simulink model "test"  (R2013a)
settings: Solver=ode45  StartTime=0.0  StopTime=time  RelTol=1e-3
values from neighbouring files (symbols this model uses):
  b = 0.1    [init.m]    (also in pathPlotter.m = 0.025)
  eta_0 = [0,0,0,0,0,0]'    [init.m]
  g = 9.81    [init.m]
  I = diag([0.1, 0.1, 0.2])    [init.m]
  k = 3    [init.m]
  K_d = diag([-1,-1,-0.5])    [init.m]
  k_d = -20    [init.m]
  K_d_pos = 2*sqrt(K_p_pos(1,1))*eye(2)    [init.m]
  K_i = diag([0,0,0])    [init.m]
  k_i = 150    [init.m]
  K_i_pos = 0.05 * eye(2)    [init.m]
  K_p = diag([20,20,0.45])    [init.m]
  k_p = 100    [init.m]
  K_p_pos = 0.5*eye(2)    [init.m]
  l = 0.25    [init.m]
  m = 3    [init.m]
  nodePosition = [0.5,0.5,0]'    [init.m]
  nu_0 = [0,0,0,0,0,0]'    [init.m]
  pos_ref = [10,10,-10]'    [init.m]
  wind = [0.5,0]'    [init.m]
  windDir = 0    [init.m]
libraries: simulink x1
settings Model: Creator=vegardvo  LastModifiedBy=vegardvo

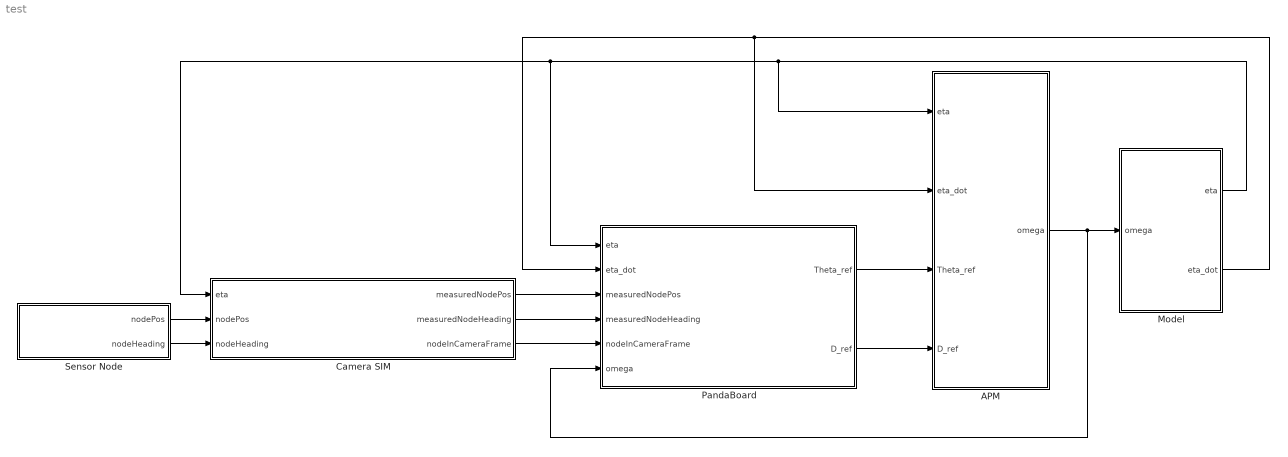
== system test ==
  APM : Subsystem
  Camera SIM : Subsystem
  Model : Subsystem
  PandaBoard : Subsystem
  Sensor Node : Subsystem
  wires:
  Sensor Node/1(nodePos) -> Camera SIM/2(nodePos)
  Sensor Node/2(nodeHeading) -> Camera SIM/3(nodeHeading)
  APM/1(omega) -> Model/1(omega), PandaBoard/6(omega)
  Model/1(eta) -> APM/1(eta), PandaBoard/1(eta), Camera SIM/1(eta)
  Model/2(eta_dot) -> APM/2(eta_dot), PandaBoard/2(eta_dot)
  Camera SIM/3(nodeInCameraFrame) -> PandaBoard/5(nodeInCameraFrame)
  Camera SIM/2(measuredNodeHeading) -> PandaBoard/4(measuredNodeHeading)
  Camera SIM/1(measuredNodePos) -> PandaBoard/3(measuredNodePos)
  PandaBoard/1(Theta_ref) -> APM/3(Theta_ref)
  PandaBoard/2(D_ref) -> APM/4(D_ref)

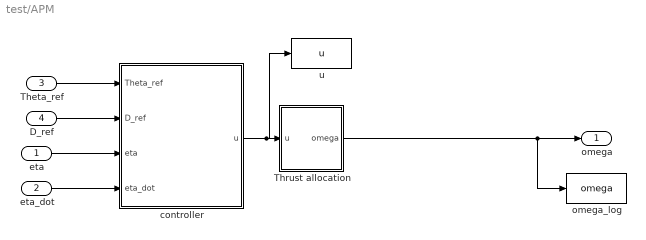
== system test/APM ==
  eta : Inport
  eta_dot : Inport  Port=2
  Theta_ref : Inport  Port=3
  D_ref : Inport  Port=4
  Thrust allocation : Subsystem
  controller : Subsystem
  omega_log : ToWorkspace  VariableName=omega  SampleTime=-1  SaveFormat=Timeseries
  u : ToWorkspace  VariableName=u  SampleTime=-1  SaveFormat=Timeseries
  omega : Outport
  wires:
  Thrust allocation/1(omega) -> omega/1, omega_log/1
  controller/1(u) -> u/1, Thrust allocation/1(u)
  D_ref/1 -> controller/2(D_ref)
  Theta_ref/1 -> controller/1(Theta_ref)
  eta/1 -> controller/3(eta)
  eta_dot/1 -> controller/4(eta_dot)

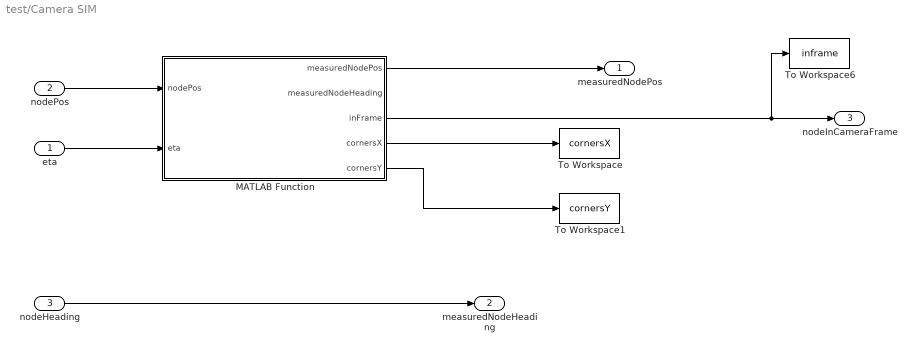
== system test/Camera SIM ==
  eta : Inport
  nodePos : Inport  Port=2
  nodeHeading : Inport  Port=3
  MATLAB Function : MATLAB Function  TreatAsAtomicUnit=on
  To Workspace : ToWorkspace  VariableName=cornersX  SampleTime=-1  SaveFormat=Timeseries
  To Workspace1 : ToWorkspace  VariableName=cornersY  SampleTime=-1  SaveFormat=Timeseries
  To Workspace6 : ToWorkspace  VariableName=inframe  SampleTime=-1  SaveFormat=Timeseries
  measuredNodePos : Outport
  measuredNodeHeading : Outport  Port=2
  nodeInCameraFrame : Outport  Port=3
  wires:
  nodePos/1 -> MATLAB Function/1(nodePos)
  MATLAB Function/1(measuredNodePos) -> measuredNodePos/1
  eta/1 -> MATLAB Function/2(eta)
  MATLAB Function/3(inFrame) -> To Workspace6/1, nodeInCameraFrame/1
  nodeHeading/1 -> measuredNodeHeading/1
  MATLAB Function/4(cornersX) -> To Workspace/1
  MATLAB Function/5(cornersY) -> To Workspace1/1

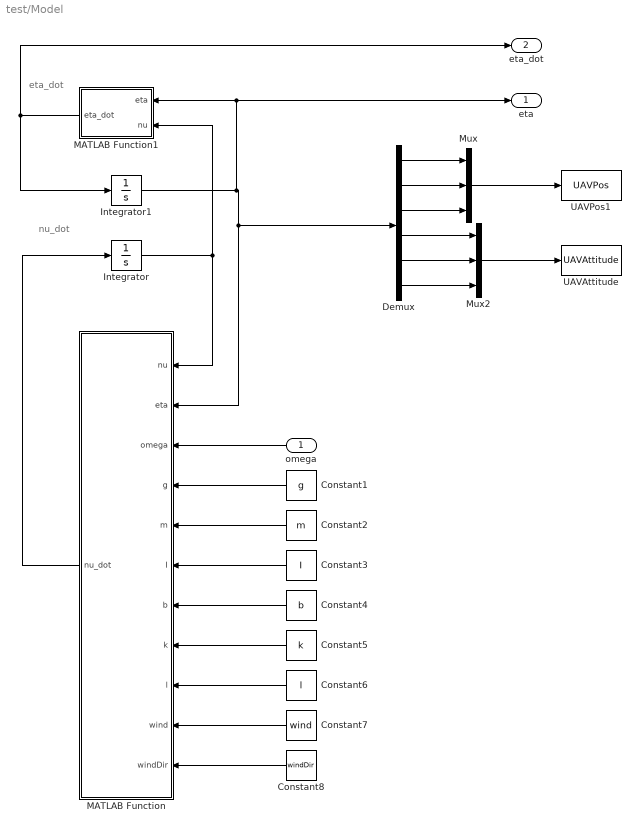
== system test/Model ==
  note: eta_dot
  note: nu_dot
  omega : Inport
  Constant1 : Constant  Value=g
  Constant2 : Constant  Value=m
  Constant3 : Constant  Value=I
  Constant4 : Constant  Value=b
  Constant5 : Constant  Value=k
  Constant6 : Constant  Value=l
  Constant7 : Constant  Value=wind
  Constant8 : Constant  Value=windDir
  Demux : Demux  Outputs=6
  Integrator : Integrator  InitialCondition=nu_0
  Integrator1 : Integrator  InitialCondition=eta_0
  MATLAB Function : MATLAB Function  TreatAsAtomicUnit=on
  MATLAB Function1 : MATLAB Function  TreatAsAtomicUnit=on
  Mux : Mux  Inputs=3
  Mux2 : Mux  Inputs=3
  UAVAttitude : ToWorkspace  VariableName=UAVAttitude  SampleTime=-1  SaveFormat=Timeseries
  UAVPos1 : ToWorkspace  VariableName=UAVPos  SampleTime=-1  SaveFormat=Timeseries
  eta : Outport
  eta_dot : Outport  Port=2
  wires:
  MATLAB Function/1(nu_dot) -> Integrator/1
  Integrator/1 -> MATLAB Function/1(nu), MATLAB Function1/2(nu)
  Integrator1/1 -> MATLAB Function/2(eta), Demux/1, MATLAB Function1/1(eta), eta/1
  Constant1/1 -> MATLAB Function/4(g)
  Constant2/1 -> MATLAB Function/5(m)
  Constant3/1 -> MATLAB Function/6(I)
  Demux/1 -> Mux/1
  Demux/2 -> Mux/2
  Demux/3 -> Mux/3
  Demux/4 -> Mux2/1
  Demux/5 -> Mux2/2
  Demux/6 -> Mux2/3
  Constant4/1 -> MATLAB Function/7(b)
  Constant5/1 -> MATLAB Function/8(k)
  Constant6/1 -> MATLAB Function/9(l)
  MATLAB Function1/1(eta_dot) -> Integrator1/1, eta_dot/1
  omega/1 -> MATLAB Function/3(omega)
  Mux/1 -> UAVPos1/1
  Mux2/1 -> UAVAttitude/1
  Constant8/1 -> MATLAB Function/11(windDir)
  Constant7/1 -> MATLAB Function/10(wind)

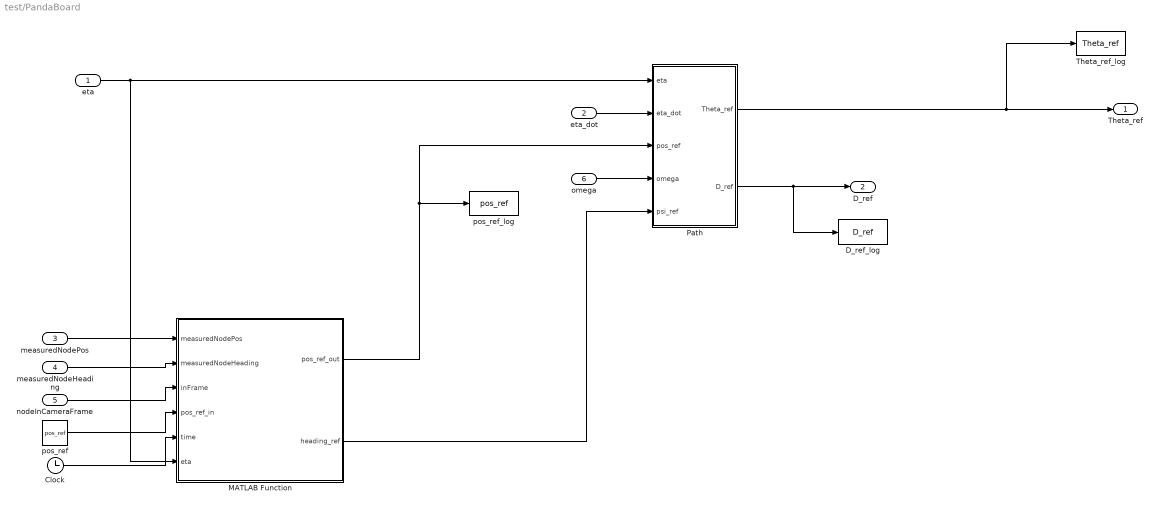
== system test/PandaBoard ==
  eta : Inport
  eta_dot : Inport  Port=2
  measuredNodePos : Inport  Port=3
  measuredNodeHeading : Inport  Port=4
  nodeInCameraFrame : Inport  Port=5
  omega : Inport  Port=6
  Clock : Clock
  D_ref_log : ToWorkspace  VariableName=D_ref  SampleTime=-1  SaveFormat=Timeseries
  MATLAB Function : MATLAB Function  TreatAsAtomicUnit=on
  Path : Subsystem
  Theta_ref_log : ToWorkspace  VariableName=Theta_ref  SampleTime=-1  SaveFormat=Timeseries
  pos_ref : Constant  Value=pos_ref
  pos_ref_log : ToWorkspace  VariableName=pos_ref  SampleTime=-1  SaveFormat=Timeseries
  Theta_ref : Outport
  D_ref : Outport  Port=2
  wires:
  Path/2(D_ref) -> D_ref/1, D_ref_log/1
  omega/1 -> Path/4(omega)
  eta_dot/1 -> Path/2(eta_dot)
  eta/1 -> MATLAB Function/6(eta), Path/1(eta)
  measuredNodePos/1 -> MATLAB Function/1(measuredNodePos)
  measuredNodeHeading/1 -> MATLAB Function/2(measuredNodeHeading)
  nodeInCameraFrame/1 -> MATLAB Function/3(inFrame)
  pos_ref/1 -> MATLAB Function/4(pos_ref_in)
  MATLAB Function/1(pos_ref_out) -> Path/3(pos_ref), pos_ref_log/1
  MATLAB Function/2(heading_ref) -> Path/5(psi_ref)
  Clock/1 -> MATLAB Function/5(time)
  Path/1(Theta_ref) -> Theta_ref_log/1, Theta_ref/1

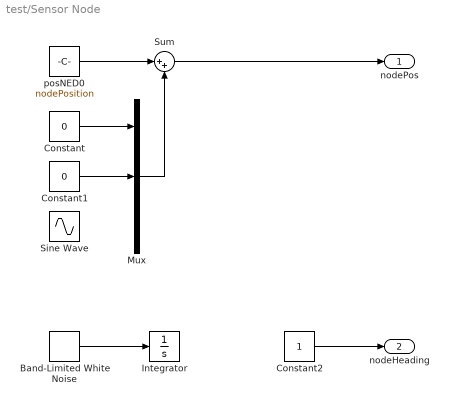
== system test/Sensor Node ==
  Band-Limited White Noise : simulink/Sources/Band-Limited White Noise  Cov=[0.1]  Ts=0.1  seed=[23341]
  Constant : Constant  Value=0
  Constant1 : Constant  Value=0
  Constant2 : Constant
  Integrator : Integrator
  Mux : Mux  Inputs=3
  Sine Wave : Sin  SampleTime=0
  Sum : Sum  Inputs=|++
  posNED0 : Constant  Value=nodePosition
  nodePos : Outport
  nodeHeading : Outport  Port=2
  wires:
  posNED0/1 -> Sum/1
  Sum/1 -> nodePos/1
  Mux/1 -> Sum/2
  Constant1/1 -> Mux/2
  Constant/1 -> Mux/1
  Band-Limited White Noise/1 -> Integrator/1
  Constant2/1 -> nodeHeading/1

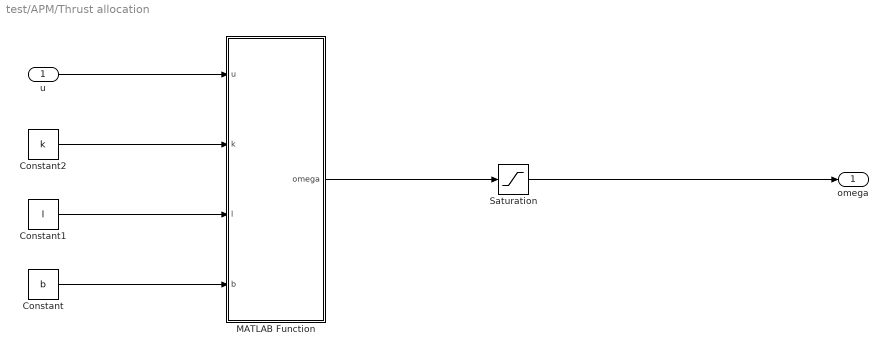
== system test/APM/Thrust allocation ==
  u : Inport
  Constant : Constant  Value=b
  Constant1 : Constant  Value=l
  Constant2 : Constant  Value=k
  MATLAB Function : MATLAB Function  TreatAsAtomicUnit=on
  Saturation : Saturate  UpperLimit=Inf  LowerLimit=0  ZeroCross=off
  omega : Outport
  wires:
  u/1 -> MATLAB Function/1(u)
  Constant2/1 -> MATLAB Function/2(k)
  Constant1/1 -> MATLAB Function/3(l)
  Constant/1 -> MATLAB Function/4(b)
  MATLAB Function/1(omega) -> Saturation/1
  Saturation/1 -> omega/1

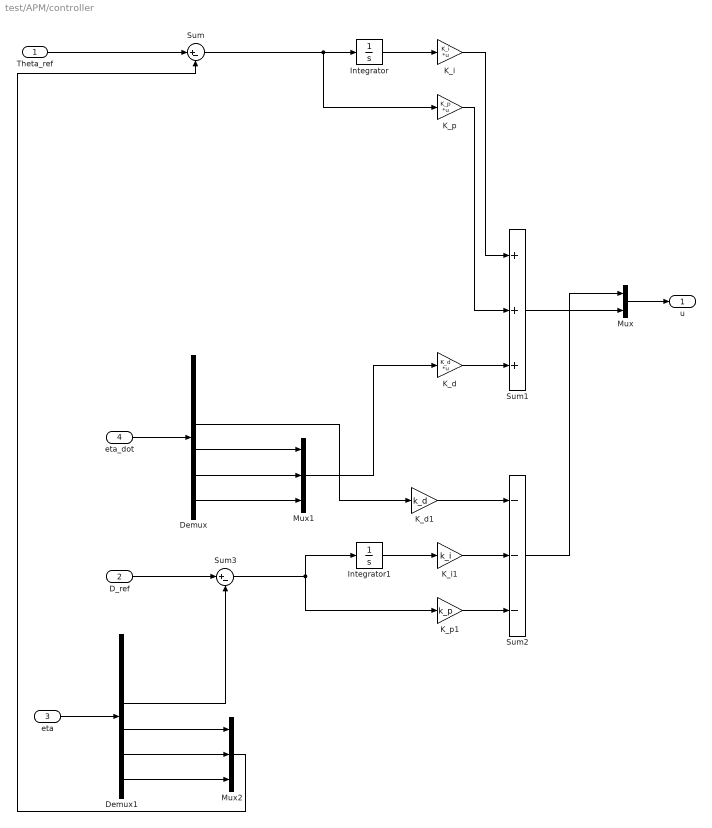
== system test/APM/controller ==
  Theta_ref : Inport
  D_ref : Inport  Port=2
  eta : Inport  Port=3
  eta_dot : Inport  Port=4
  Demux : Demux  Outputs=6
  Demux1 : Demux  Outputs=6
  Integrator : Integrator  InitialCondition=[0,0,0]'
  Integrator1 : Integrator
  K_d : Gain  Gain=K_d  Multiplication=Matrix(K*u)
  K_d1 : Gain  Gain=k_d
  K_i : Gain  Gain=K_i  Multiplication=Matrix(K*u)
  K_i1 : Gain  Gain=k_i
  K_p : Gain  Gain=K_p  Multiplication=Matrix(K*u)
  K_p1 : Gain  Gain=k_p
  Mux : Mux  Inputs=2
  Mux1 : Mux  Inputs=3
  Mux2 : Mux  Inputs=3
  Sum : Sum  Inputs=|+-
  Sum1 : Sum  Inputs=+++
  Sum2 : Sum  Inputs=---
  Sum3 : Sum  Inputs=|+-
  u : Outport
  wires:
  Sum/1 -> K_p/1, Integrator/1
  Integrator/1 -> K_i/1
  K_i/1 -> Sum1/1
  K_p/1 -> Sum1/2
  K_d/1 -> Sum1/3
  Integrator1/1 -> K_i1/1
  D_ref/1 -> Sum3/1
  Sum3/1 -> K_p1/1, Integrator1/1
  Mux/1 -> u/1
  eta_dot/1 -> Demux/1
  Mux1/1 -> K_d/1
  K_d1/1 -> Sum2/1
  eta/1 -> Demux1/1
  K_i1/1 -> Sum2/2
  K_p1/1 -> Sum2/3
  Sum2/1 -> Mux/1
  Sum1/1 -> Mux/2
  Demux1/3 -> Sum3/2
  Demux1/4 -> Mux2/1
  Demux1/5 -> Mux2/2
  Demux1/6 -> Mux2/3
  Mux2/1 -> Sum/2
  Demux/4 -> Mux1/1
  Demux/5 -> Mux1/2
  Demux/6 -> Mux1/3
  Demux/3 -> K_d1/1
  Theta_ref/1 -> Sum/1

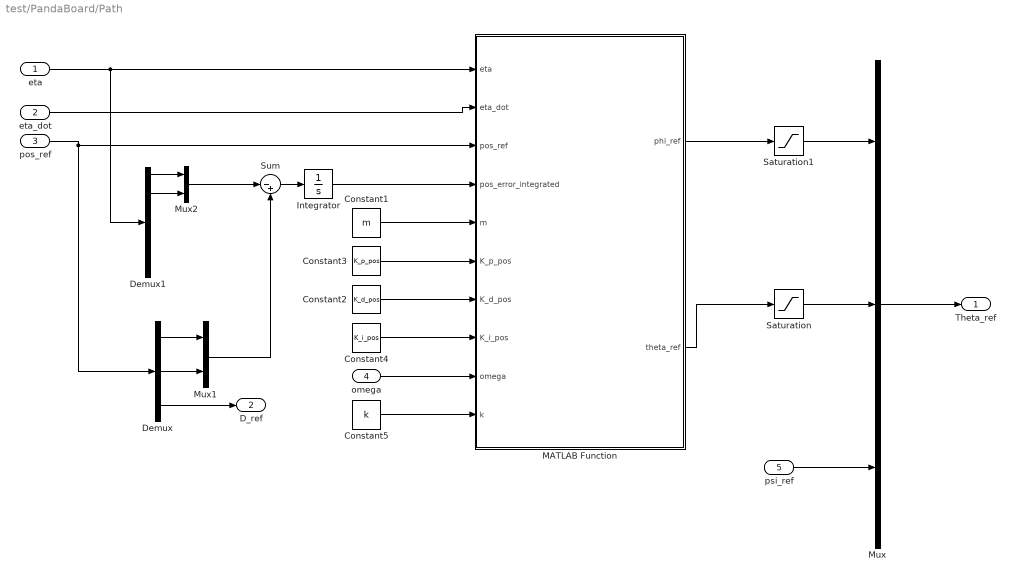
== system test/PandaBoard/Path ==
  eta : Inport
  eta_dot : Inport  Port=2
  pos_ref : Inport  Port=3
  omega : Inport  Port=4
  psi_ref : Inport  Port=5
  Constant1 : Constant  Value=m
  Constant2 : Constant  Value=K_d_pos
  Constant3 : Constant  Value=K_p_pos
  Constant4 : Constant  Value=K_i_pos
  Constant5 : Constant  Value=k
  Demux : Demux  Outputs=3
  Demux1 : Demux  Outputs=6
  Integrator : Integrator  LimitOutput=on  UpperSaturationLimit=100  LowerSaturationLimit=-100
  MATLAB Function : MATLAB Function  TreatAsAtomicUnit=on
  Mux : Mux  Inputs=3
  Mux1 : Mux  Inputs=2
  Mux2 : Mux  Inputs=2
  Saturation : Saturate  UpperLimit=0.2  LowerLimit=-0.2  ZeroCross=off
  Saturation1 : Saturate  UpperLimit=0.2  LowerLimit=-0.2  ZeroCross=off
  Sum : Sum  Inputs=|-+
  Theta_ref : Outport
  D_ref : Outport  Port=2
  wires:
  Mux/1 -> Theta_ref/1
  eta/1 -> Demux1/1, MATLAB Function/1(eta)
  pos_ref/1 -> MATLAB Function/3(pos_ref), Demux/1
  Demux/3 -> D_ref/1
  eta_dot/1 -> MATLAB Function/2(eta_dot)
  Constant1/1 -> MATLAB Function/5(m)
  Constant3/1 -> MATLAB Function/6(K_p_pos)
  Constant2/1 -> MATLAB Function/7(K_d_pos)
  MATLAB Function/1(phi_ref) -> Saturation1/1
  MATLAB Function/2(theta_ref) -> Saturation/1
  Saturation1/1 -> Mux/1
  Saturation/1 -> Mux/2
  psi_ref/1 -> Mux/3
  omega/1 -> MATLAB Function/9(omega)
  Constant5/1 -> MATLAB Function/10(k)
  Constant4/1 -> MATLAB Function/8(K_i_pos)
  Integrator/1 -> MATLAB Function/4(pos_error_integrated)
  Sum/1 -> Integrator/1
  Demux/1 -> Mux1/1
  Demux/2 -> Mux1/2
  Demux1/1 -> Mux2/1
  Demux1/2 -> Mux2/2
  Mux2/1 -> Sum/1
  Mux1/1 -> Sum/2

== matlab function test/APM/Thrust allocation/MATLAB Function ==
  data: u input; omega output; k input; l input; b input
function omega = fcn(u, k, l, b)
%#codegen

A = [k, k, k, k, k, k;
     -0.5*k*l, 0.5*k*l, k*l, 0.5*k*l, -0.5*k*l, -k*l;
     sqrt(3)/2*k*l, sqrt(3)/2*k*l, 0, -sqrt(3)/2*k*l, -sqrt(3)/2*k*l, 0;
     b, -b, b, -b, b, -b];

 A_pseudo = A'/(A*A');

omega = A_pseudo*u;
%omega = [1,1,1,1,1,1]';

== matlab function test/Model/MATLAB Function ==
  data: nu input; nu_dot output; eta input; omega input; g input; m input; I input; b input; k input; l input; wind input; windDir input
function nu_dot = fcn(nu, eta, omega, g, m, I, b, k, l, wind, windDir)
%#codegen

omega_squared = omega;%omega.^2;

M_rb = [m * eye(3), zeros(3);
        zeros(3)  , I];
 
%C_rb = [m*Smtrx(nu(4:6)), zeros(3);
%       zeros(3), -Smtrx(I*nu(4:6))];
   
C_rb = m2c(M_rb, nu);

RotWind = [cos(windDir), sin(windDir);
          -sin(windDir), cos(windDir)];
wind_b = RotWind * wind;

tau_b = [-m*g*sin(eta(5)) + wind_b(1);
       m*g*cos(eta(5))*sin(eta(4)) + wind_b(2);
       m*g*cos(eta(5))*cos(eta(4)) - k*sum(omega_squared);
       k*l*[-0.5, 0.5, 1, 0.5, -0.5, -1]*omega_squared;
       sqrt(3)/2 * k *l * [1,1,0,-1,-1,0]*omega_squared;
       b*[1,-1,1,-1,1,-1]*omega_squared];

nu_dot = M_rb\(tau_b - C_rb*nu);

== matlab function test/Model/MATLAB Function1 ==
  data: eta input; eta_dot output; nu input
function eta_dot = fcn(eta, nu)
%#codegen

[J, J11, J22] = eulerang(eta(4), eta(5), eta(6));

eta_dot = J*nu;

== matlab function test/PandaBoard/Path/MATLAB Function ==
  data: eta input; eta_dot input; phi_ref output; pos_ref input; pos_error_integrated input; theta_ref output; m input; K_p_pos input; K_d_pos input; K_i_pos input; omega input; k input
function [phi_ref, theta_ref]= fcn(eta,eta_dot, pos_ref, pos_error_integrated, m, K_p_pos, K_d_pos, K_i_pos, omega, k)
%#codegen
% 
psi = eta(6);
T = k*sum(omega);
if T==0
    T = 0.1;
end
B_inv = m/T * [-sin(psi), cos(psi);
               -cos(psi), -sin(psi)]; %OBS SINGULARITET
Theta_ref = B_inv*(-K_d_pos*eta_dot(1:2) - K_p_pos*eta(1:2) + K_p_pos*pos_ref(1:2) + K_i_pos * pos_error_integrated);
theta_ref = Theta_ref(2);
phi_ref = Theta_ref(1);

%theta_ref = 1/g*(k_d_pos * eta_dot(1) - k_p_pos*(pos_ref(1)-eta(1)));
%phi_ref = 1/g*(-k_d_pos * eta_dot(2) + k_p_pos*(pos_ref(2)-eta(2)));

== matlab function test/Camera SIM/MATLAB Function ==
  data: nodePos input; measuredNodePos output; measuredNodeHeading output; eta input; inFrame output; cornersX output; cornersY output
function [measuredNodePos, measuredNodeHeading, inFrame, cornersX, cornersY] = fcn(nodePos, eta)
%#codegen


% Calculate area where camera active
	% Init variables
    x_c = 320;
    y_c = 240;
    
    phi = eta(4);
    theta = eta(5);
    psi = eta(6);
    height = eta(3);
    
    d1 = 0;
    lengthPerPixel = 0.001328497723204;
    
    sinPhi = sin(phi);
	cosPhi = cos(phi);

	sinTheta = sin(theta);
	cosTheta = cos(theta);

	sinPsi = sin(psi);
	cosPsi = cos(psi);
    

    
    
    corners = zeros(4,2);
    x = 0;
    y = 0;
    for i = 1:4
        switch(i)
            case 1
                x = 0;
                y = 0;
            case 2
                x = 640;
                y = 0;
            case 3
                x = 640;
                y = 480;
            case 4
                x = 0;
                y = 480;
        end;
    
    deltaX = x - x_c;
 	deltaY = y - y_c;
   
    alpha = -atan2(-deltaY, deltaX);
 	d = sqrt(deltaX^2 + deltaY^2) * lengthPerPixel;
 	beta = -atan(d);
    
 	sinAlpha = sin(alpha);
 	cosAlpha = cos(alpha);
 	sinBeta = sin(beta);
 	cosBeta = cos(beta);
    
    z1 = cosPsi * cosTheta * sinAlpha * sinBeta - cosAlpha * sinBeta * (-sinPsi * cosPhi + cosPsi * sinTheta * sinPhi) + cosBeta * (sinPsi * sinPhi + cosPsi * sinTheta * cosPhi);
    z2 = sinPsi * cosTheta * sinAlpha * sinBeta - cosAlpha * sinBeta * (cosPsi * cosPhi + sinPsi * sinTheta * sinPhi) + cosBeta * (-cosPsi * sinPhi + sinPsi *sinTheta *cosPhi);
    z3 = -sinTheta * sinAlpha * sinBeta - cosAlpha * sinBeta * cosTheta * sinPhi + cosBeta * cosTheta * cosPhi;
    
    d2 = (abs(height) - d1*cosTheta*cosPhi)/z3; %OBS ABS
    
 	corners(i,1) = d2*z1 + d1*(sinPsi*sinPhi + cosPsi*sinTheta*cosPhi) + eta(1);
 	corners(i,2) = d2*z2 + d1*(-cosPsi*sinPhi + sinPsi*sinTheta*cosPhi) + eta(2);    
    end;
    result = false;
    j = 4;
for i = 1:4
    if ((corners(i,2) > nodePos(2)) ~= (corners(j,2) > nodePos(2)) && (nodePos(1) < (corners(j,1) - corners(i,1))*(nodePos(2) - corners(i,2))/(corners(j,2)-corners(i,2))+corners(i,1)))
        result = ~result;
    end
    j = i;
end
measuredNodePos = nodePos; 
measuredNodeHeading = 1;
inFrame = result;
cornersX = corners(:, 1);
cornersY = corners(:, 2);

== matlab function test/PandaBoard/MATLAB Function ==
  data: measuredNodePos input; pos_ref_out output; measuredNodeHeading input; inFrame input; heading_ref output; pos_ref_in input; time input; eta input
function [pos_ref_out, heading_ref]= fcn(measuredNodePos, measuredNodeHeading, inFrame, pos_ref_in, time, eta)
%#codegen

persistent heading;

if isempty(heading)
     heading = 0;
end
pos_ref_out = [0;0;pos_ref_in(3)];
if inFrame == 1
    pos_ref_out(1) = measuredNodePos(1);
    pos_ref_out(2) = measuredNodePos(2);
    %pos_ref_out(3) = measuredNodePos(3);
    heading = measuredNodeHeading;
else
    pos_ref_out(1) = eta(1);
    pos_ref_out(2) = eta(2);
    %pos_ref_out(3) = pos_ref_in(3);

end
    heading_ref = heading;

% Ramp up height
 persistent timeLastCycle;
 if isempty(timeLastCycle)
     timeLastCycle = 0;
 end
 timeStep = time - timeLastCycle;
 timeLastCycle = time;
 
 persistent lastDesHeight;
 if isempty(lastDesHeight)
     lastDesHeight = 0;
 end

% % Hardkodet med 0.25 m/s og 1.5 m som referanse - Tja
 
     pos_ref_out(3) = lastDesHeight - 0.25 * 4 * timeStep;
     lastDesHeight = pos_ref_out(3);

     if pos_ref_out(3) < -4
        pos_ref_out(3) = -4;
        lastDesHeight = pos_ref_out(3);
     end
     
     if sqrt((eta(1)-measuredNodePos(1))^2 + (eta(2)-measuredNodePos(2))^2) < 0.05 && inFrame == 1
        pos_ref_out(3) = lastDesHeight + 0.25 * timeStep;
        lastDesHeight = pos_ref_out(3);
        if pos_ref_out(3) > -0.05
            pos_ref_out(3) = -0.05;
            lastDesHeight = pos_ref_out(3);

        end
     else
         pos_ref_out(3) = lastDesHeight;
     end
